simulink model "UAVUGV"  (R2018a)
settings: Solver=VariableStepAuto  StartTime=0.0  StopTime=300  RelTol=1e-3
libraries: simulink x1
settings Model: Creator=wangluo  LastModifiedBy=wangluo

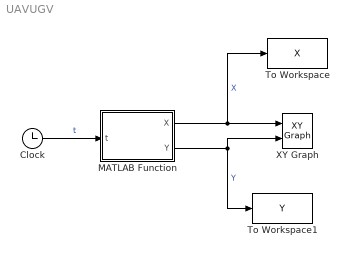
== system UAVUGV ==
  Clock : Clock
      settings: Decimation=300
  MATLAB Function : MATLAB Function  TreatAsAtomicUnit=on
  To Workspace : ToWorkspace  VariableName=X  SaveFormat=Timeseries  SampleTime=-1
  To Workspace1 : ToWorkspace  VariableName=Y  SaveFormat=Timeseries  SampleTime=-1
  XY Graph : simulink/Sinks/XY Graph  xmin=-10  xmax=20  ymin=-10  ymax=15  st=-1
  wires:
  MATLAB Function/1(X) -> To Workspace/1, XY Graph/1  "X"
  Clock/1 -> MATLAB Function/1(t)  "t"
  MATLAB Function/2(Y) -> To Workspace1/1, XY Graph/2  "Y"

== matlab function UAVUGV/MATLAB Function ==
  data: t input; X output; Y output
function [X, Y] = fcn(t)
% #codegen

% calculates a statistical mean and a standard
% deviation for the values in vals

i=0;
j=0;
X = 0;
Y = 0;

% Leader Trajectory
if (0<=t)&&(t<=30)
    i = i + 1; j = j + 1;
    X(:,i) = -8;
    Y(:,j) = t/6 - 8;
    
elseif (30<=t)&&(t<=60)
    i = i + 1; j = j + 1;
    X(:,i) = (t-30)/6 - 8;
    Y(:,j) = -3;
    
elseif (60<=t)&&(t<=90)
    i = i + 1; j = j + 1;
    X(:,i) = (t-60)/10 - 3;
    Y(:,j) = (t-60)/10 - 3;
    
elseif (90<=t)&&(t<=120)
    i = i + 1; j = j + 1;
    X(:,i) = 0;
    Y(:,j) = (t-90)/3;
    
elseif (120<=t)&&(t<=150)
    i = i + 1; j = j + 1;
    X(:,i) = (t-120)/10;
    Y(:,j) = (t-120)/10 + 10;
    
elseif (150<=t)&&(t<=180)
    i = i + 1; j = j + 1;
    X(:,i) = (t-150)/6 + 3;
    Y(:,j) = 13;
    
elseif (180<=t)&&(t<=210)
    i = i + 1; j = j + 1;
    X(:,i) = (t-180)/6 + 8;
    Y(:,j) = (t-180)/(-10) + 13;

elseif (210<=t)&&(t<=240)
    i = i + 1; j = j + 1;
    X(:,i) = 13;
    Y(:,j) = (t-210)/(-3) + 10;

elseif (240<=t)&&(t<=270)
    i = i + 1; j = j + 1;
    X(:,i) = (t-240)/6 + 13;
    Y(:,j) = (t-240)/(-10); 
    
elseif (270<=t)&&(t<=300)
    i = i + 1; j = j + 1;
    X(:,i) = (t-210)/15+18;
    Y(:,j) = -3;
end
